simulink model "testArgosModel"  (R2018b)
settings: Solver=FixedStepAuto  StartTime=0.0  StopTime=10.0  RelTol=1e-3
settings Model: Creator=sebastian  LastModifiedBy=sebastian
settings OptimizationCC: DefaultParameterBehavior=Inlined  EnhancedBackFolding=on  PassReuseOutputArgsAs=Individual arguments  ZeroExternalMemoryAtStartup=off  OptimizeBlockOrder=speed  DifferentSizesBufferReuse=on  OptimizationCustomize=off
settings DebuggingCC: ParameterTunabilityLossMsg=error
settings SFSimCC: MATLABDynamicMemAlloc=off
settings RTWCC: SystemTargetFile=ert.tlc  GenCodeOnly=on  PackageName=testZip  TemplateMakefile=ert_default_tmf  PostCodeGenCommand=exportARGoSCode(modelName,buildInfo)  GenerateReport=on  IncludeHyperlinkInReport=on  LaunchReport=on  TargetLang=C++  GenerateTraceInfo=on  GenerateTraceReport=on  GenerateTraceReportSl=on  GenerateTraceReportSf=on  GenerateTraceReportEml=on
settings CodeAppCC: ForceParamTrailComments=on  IgnoreCustomStorageClasses=off  OperatorAnnotations=on  SimulinkDataObjDesc=on  SFDataObjDesc=on  InsertBlockDesc=on
settings ERTTargetCC: TargetLangStandard=C++03 (ISO)  GenerateSampleERTMain=on  MultiInstanceERTCode=on  CodeInterfacePackaging=C++ class  SupportVariableSizeSignals=on  InlinedParameterPlacement=NonHierarchical  RootIOFormat=Structure reference  ERTCustomFileTemplate=example_file_process.tlc

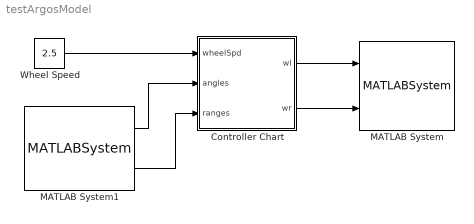
== system testArgosModel ==
  Controller Chart : Stateflow chart  TreatAsAtomicUnit=on
  MATLAB System : MATLABSystem  System=ARGoSDifferentialSteering  SimulateUsing=Interpreted execution
      mask Type: ARGoSDifferentialSteering
      mask Display:
      | disp(['ARGoS' char(10) 'Differential' char(10) 'Steering']);
      | port_label('input',1,'wl');
      | port_label('input',2,'wr');
  MATLAB System1 : MATLABSystem  System=ARGoSFootBotProximitySensor  numReadings=25  SimulateUsing=Interpreted execution
      mask Type: ARGoSFootBotProximitySensor
      mask Display:
      | disp(['ARGoS' char(10) 'FootBot' char(10) 'Proximity']);
      | port_label('output',1,'angles');
      | port_label('output',2,'ranges');
  Wheel Speed : Constant  Value=2.5
  wires:
  Controller Chart/1(wl) -> MATLAB System/1
  Controller Chart/2(wr) -> MATLAB System/2
  Wheel Speed/1 -> Controller Chart/1(wheelSpd)
  MATLAB System1/1 -> Controller Chart/2(angles)
  MATLAB System1/2 -> Controller Chart/3(ranges)

== stateflow chart testArgosModel/Controller Chart ==
  state Main
    en, du:
    validIdx = ranges>0;
    numValid = numel(validIdx);
    avgAng = sum(angles(validIdx))/numValid;
    state Straight
      en:
      wl = wheelSpd;
      wr = wheelSpd;
    state Turn
      state TurnLeft
        en:
        wl = 0;
        wr = wheelSpd;
      state TurnRight
        en:
        wl = wheelSpd;
        wr = 0;
      (default) -> (junction 12)
      (junction 12) -> TurnRight [order 2]
      (junction 12) -> TurnLeft [order 1] : [avgAng<0]
      TurnLeft -> TurnRight : [avgAng > 0]
      TurnRight -> TurnLeft : [avgAng < 0]
    (default) -> Straight
    Straight -> Turn : [~isClear() && ...
        |    numValid > 0]
    Turn -> Straight : [isClear || ...
        |  numValid == 0]
  state out = isClear [function]
    (default) -> (junction 29) : % Checks if clear to go straight
        | {
        | out = ...
        | all(angles(validIdx) <= deg2rad(10)) && ...
        | all(ranges(validIdx) >= 0.5);
        | }
  (default) -> Main
  data: out function_output; wl output; wr output; wheelSpd input; angles input; ranges input; validIdx local; numValid local; avgAng local
